simulink model "SingleJointedArm"  (R2022a)
settings: Solver=VariableStepAuto  StartTime=0.0  StopTime=10.0  RelTol=1e-3
values from neighbouring files (symbols this model uses):
  A = zeros(2)    [InvertedPendulum.m]    (also in RunSingleJointedArm.m = [0, 1)
  B = -eye(2)/Ts    [InvertedPendulum.m]    (also in RunSingleJointedArm.m = [0)
  C = [0 0; 1 0; 0 0; 0 1]    [InvertedPendulum.m]    (also in RunSingleJointedArm.m = eye(2))
  D = [1 0; 1/Ts 0; 0 1; 0 1/Ts]    [InvertedPendulum.m]    (also in RunSingleJointedArm.m = [0; 0])
  K = [0 -18 -166.5 -15.2]    [InvertedPendulum.m]    (also in RunSingleJointedArm.m = place(A, B, poles))
settings Model: Creator=woz4t  LastModifiedBy=woz4t

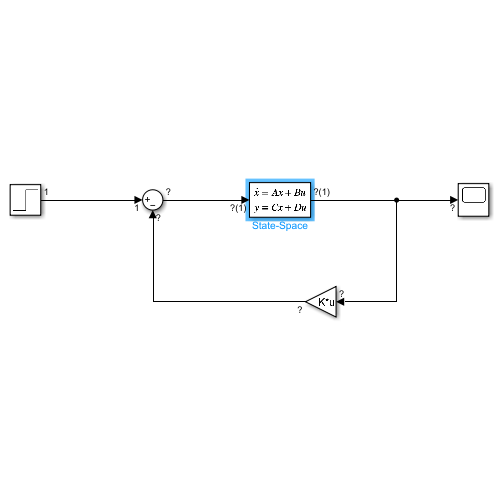
[thumbnail: Simulink's stored preview of the top-level diagram]
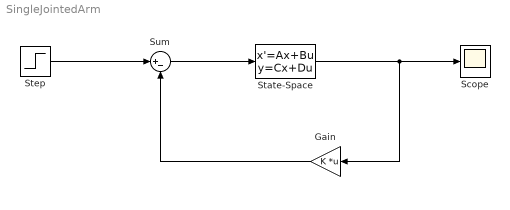
== system SingleJointedArm ==
  Gain : Gain  Gain=K  Multiplication=Matrix(K*u)
  Scope : Scope
  State-Space : StateSpace  A=A  B=B  C=C  D=D  InitialCondition=0
  Step : Step  SampleTime=0
  Sum : Sum  Inputs=|+-
  wires:
  State-Space/1 -> Gain/1, Scope/1
  Step/1 -> Sum/1
  Sum/1 -> State-Space/1
  Gain/1 -> Sum/2
